simulink model "PlantModel"  (R2024b)
settings: Solver=VariableStepAuto  StartTime=0.0  StopTime=200  RelTol=1e-3
model workspace (MAT data in the model file):
  Drag_Constants = 1
  mass = [5.51 5.51 5.51 1 1 1]
  mass_6a = [5 5 5 1 1 1]
settings Model: Creator=zenyn  LastModifiedBy=zenyn
settings DebuggingCC: UnderSpecifiedDimensionMsg=warning

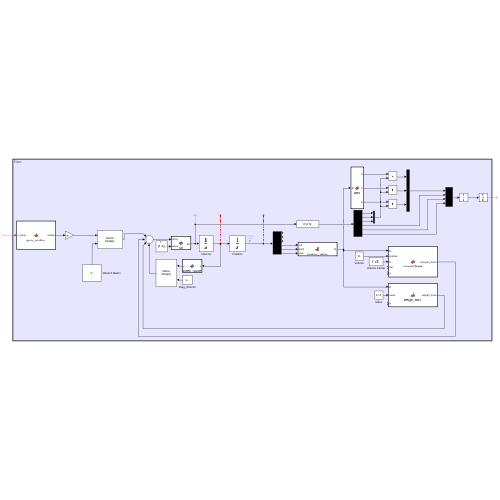
[thumbnail: Simulink's stored preview of the top-level diagram]
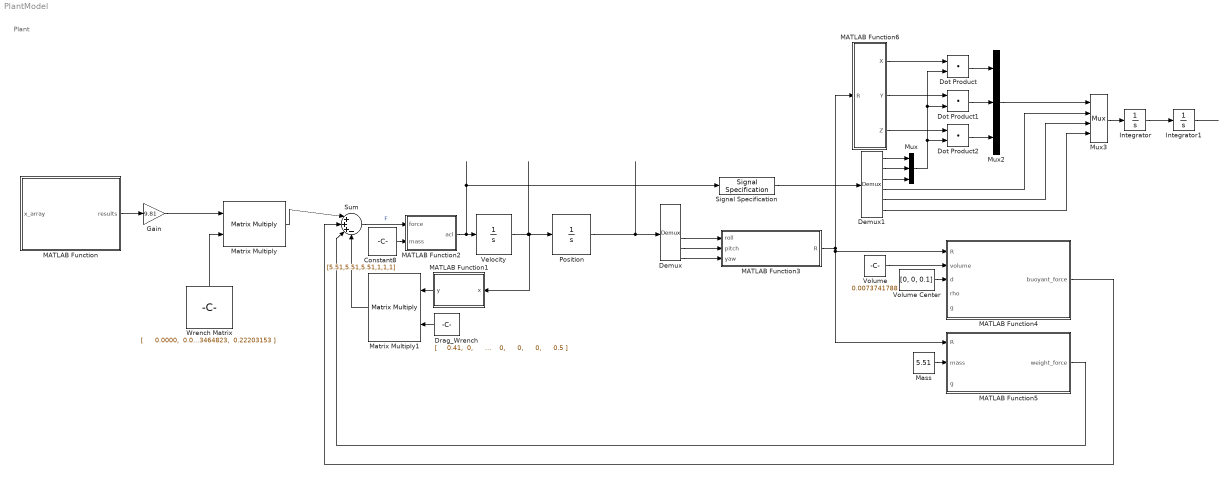
== system PlantModel ==
  note: Plant
  Constant8 : Constant  Value=[5.51,5.51,5.51,1,1,1]  VectorParams1D=off
  Demux : Demux  Outputs=6
  Demux1 : Demux  Outputs=6
  Dot Product : DotProduct  OutDataTypeStr=Inherit: Inherit via internal rule
  Dot Product1 : DotProduct  OutDataTypeStr=Inherit: Inherit via internal rule
  Dot Product2 : DotProduct  OutDataTypeStr=Inherit: Inherit via internal rule
  Drag_Wrench : Constant  Value=|  VectorParams1D=off
      | [
      |     0.41,  0,      0,      0,      0,      0;
      |     0,      0.5,   0,      0,      0,      0;
      |     0,      0,      1.25,  0,      0,      0;
      |     0,      0,      0,      0.5,   0,      0;
      |     0,      0,      0,      0,      1,    0;
      |     0,      0,      0,      0,      0,      0.5
      | ]
  Gain : Gain  Gain=9.81
  Integrator : Integrator
  Integrator1 : Integrator
  MATLAB Function : MATLAB Function  TreatAsAtomicUnit=on
  MATLAB Function1 : MATLAB Function  TreatAsAtomicUnit=on
  MATLAB Function2 : MATLAB Function  TreatAsAtomicUnit=on
  MATLAB Function3 : MATLAB Function  TreatAsAtomicUnit=on
  MATLAB Function4 : MATLAB Function  TreatAsAtomicUnit=on
  MATLAB Function5 : MATLAB Function  TreatAsAtomicUnit=on
  MATLAB Function6 : MATLAB Function  TreatAsAtomicUnit=on
  Mass : Constant  Value=5.51
  Matrix Multiply : Product  Multiplication=Matrix(*)
  Matrix Multiply1 : Product  Multiplication=Matrix(*)
  Mux : Mux  Inputs=3
  Mux2 : Mux  Inputs=3
  Mux3 : Mux
  Position : Integrator
  Signal Specification : SignalSpecification  Dimensions=[1 6]
  Sum : Sum  Inputs=|+++-
  Velocity : Integrator
  Volume : Constant  Value=0.0073741788
  Volume Center : Constant  Value=[0, 0, 0.1]
  Wrench Matrix : Constant  Value=|  VectorParams1D=off
      | [
      |      0.0000,  0.0000,  1.0000, -0.2035, -0.2535,  0.0000;
      |      0.0000,  0.0000,  1.0000,  0.2035, -0.2535,  0.0000;
      |      0.0000,  0.0000,  1.0000, -0.2035,  0.2545,  0.0000;
      |      0.0000,  0.0000,  1.0000,  0.2035,  0.2545,  0.0000;
      |     -0.7071, -0.7071,  0.0000, -0.03464823,  0.03464823, -0.21531401;
      |     -0.7071,  0.7071,  0.0000,  0.03464823,  0.03464823,  0.21531401;
      |     -0.7071,  0.7071,  0.0000,  0.03464823,  0.03464823, -0.22203153;
      |     -0.7071, -0.7071,  0.0000, -0.03464823,  0.03464823,  0.22203153
      | ]
  wires:
  Integrator1/1 -> ?
  Demux1/6 -> Mux3/4
  Demux1/5 -> Mux3/3
  Mux3/1 -> Integrator/1
  Demux1/4 -> Mux3/2
  Mux2/1 -> Mux3/1
  Dot Product2/1 -> Mux2/3
  Dot Product1/1 -> Mux2/2
  Dot Product/1 -> Mux2/1
  MATLAB Function6/3(Z) -> Dot Product2/1
  MATLAB Function6/2(Y) -> Dot Product1/1
  MATLAB Function6/1(X) -> Dot Product/1
  Mux/1 -> Dot Product2/2, Dot Product1/2, Dot Product/2
  Demux1/1 -> Mux/1
  Demux1/2 -> Mux/2
  Demux1/3 -> Mux/3
  Signal Specification/1 -> Demux1/1
  Gain/1 -> Matrix Multiply/1
  MATLAB Function4/1(buoyant_force) -> Sum/2
  Matrix Multiply/1 -> Sum/1
  Integrator/1 -> Integrator1/1
  ? -> MATLAB Function/1(x_array)
  Matrix Multiply1/1 -> Sum/4
  Demux/5 -> MATLAB Function3/2(pitch)
  MATLAB Function2/1(acl) -> Signal Specification/1, Velocity/1
  MATLAB Function3/1(R) -> MATLAB Function5/1(R), MATLAB Function4/1(R), MATLAB Function6/1(R)
  Wrench Matrix/1 -> Matrix Multiply/2
  Position/1 -> Demux/1
  Mass/1 -> MATLAB Function5/2(mass)
  MATLAB Function/1(results) -> Gain/1
  Velocity/1 -> Position/1, MATLAB Function1/1(x)
  Constant8/1 -> MATLAB Function2/2(mass)
  MATLAB Function5/1(weight_force) -> Sum/3
  MATLAB Function1/1(y) -> Matrix Multiply1/1
  Demux/6 -> MATLAB Function3/3(yaw)
  Drag_Wrench/1 -> Matrix Multiply1/2
  Sum/1 -> MATLAB Function2/1(force)  "F"
  Volume Center/1 -> MATLAB Function4/3(d)
  Volume/1 -> MATLAB Function4/2(volume)
  Demux/4 -> MATLAB Function3/1(roll)

== matlab function PlantModel/MATLAB Function1 ==
  data: x input; y output
function y = signed_square(x)
y = x .* abs(x);
end

== matlab function PlantModel/MATLAB Function ==
  data: x_array input; results output
function results = pwm_function(x_array)
    % Preallocate results array
    results = zeros(size(x_array)); 
    
    % First condition: 1100 <= x < 1460
    idx = (x_array >= 1100 & x_array < 1460);
    results(idx) = (-1.24422882971549e-8) * x_array(idx).^3 ...
                 + (4.02057100632393e-5) * x_array(idx).^2 ...
                 - 0.0348619861030835 * x_array(idx) ...
                 + 3.90671429105423;
    
    % Second condition: 1460 <= x <= 1540
    idx = (x_array >= 1460 & x_array <= 1540);
    results(idx) = 0;
    
    % Third condition: 1540 < x <= 1900
    idx = (x_array > 1540 & x_array <= 1900);
    results(idx) = (-1.64293565374284e-8) * x_array(idx).^3 ...
                 + (9.45962838560648e-5) * x_array(idx).^2 ...
                 - 0.170812079190679 * x_array(idx) ...
                 + 98.7232373648272;
    
    % Handle out-of-range values
    if any(isnan(results))
        error('Some values in x_array are out of the valid range [1100..1900].');
    end
end

== matlab function PlantModel/MATLAB Function2 ==
  data: force input; acl output; mass input
function acl = fcn(force, mass)
acl = force ./ mass;

end

== matlab function PlantModel/MATLAB Function3 ==
  data: roll input; R output; pitch input; yaw input
function R = rotation_matrix(roll, pitch, yaw)
    % Rotation matrix around X-axis (roll)
    Rx = [
        1,  0,           0;
        0,  cos(roll),  -sin(roll);
        0,  sin(roll),   cos(roll)
    ];

    % Rotation matrix around Y-axis (pitch)
    Ry = [
        cos(pitch),  0,  sin(pitch);
        0,           1,  0;
       -sin(pitch),  0,  cos(pitch)
    ];

    % Rotation matrix around Z-axis (yaw)
    Rz = [
        cos(yaw), -sin(yaw),  0;
        sin(yaw),  cos(yaw),  0;
        0,         0,         1
    ];

    % Combine rotations: R = Rz * Ry * Rx
    R = Rz * Ry * Rx;
end

== matlab function PlantModel/MATLAB Function4 ==
  data: R input; buoyant_force output; volume input; d input; rho input; g input
function buoyant_force = buoyant_force(R, volume, d, rho, g)
    % Set default values for fluid density and gravity if not provided
    if nargin < 6
        rho = 1000; % Default fluid density (kg/m³) for water
    end
    if nargin < 7
        g = 9.81; % Default gravitational acceleration (m/s²)
    end

    % Ensure d is a column vector
    d = d(:);

    % Buoyant force vector in world frame
    b_vector = [0; 0; rho * g * volume];

    % Rotate buoyant force to object's frame
    buoyant_force_body = R * b_vector;

    % Compute torque using cross product τ = d × F_buoyancy
    % (MATLAB cross function works for column vectors)
    torque = cross(-d, buoyant_force_body);

    % Combine force and torque into a single output vector
    buoyant_force = [buoyant_force_body; torque]';
end

== matlab function PlantModel/MATLAB Function5 ==
  data: R input; weight_force output; mass input; g input
function weight_force = weight_force(R, mass, g)
    % Set default gravitational acceleration if not provided
    if nargin < 4
        g = 9.81; % Default gravitational acceleration (m/s²)
    end

    % Gravity force vector in world frame (downward)
    g_vector = [0; 0; -mass * g];
    
    % Linear Force
    lin = R * g_vector;
    % Rotational force
    rot = [0;0;0];
    % Transform gravity force to rotated frame
    weight_force = [lin', rot'];
end

== matlab function PlantModel/MATLAB Function6 ==
  data: R input; X output; Y output; Z output
function [X, Y, Z] =  axes(R)
% in this function, x, y and z axes refer to direction relative current
% orientation of robot

% X, Y and Z axes refer to direction relative to intial orientation of
% robot

x_vector = [1; 0; 0];
y_vector = [0; 1; 0];
z_vector = [0; 0; 1];

X = [R * x_vector];
Y = [R * y_vector];
Z = [R * z_vector];

end
